simulink model "lab2_pogonya_2018b"  (R2018b)
settings: Solver=FixedStepAuto  StartTime=0.0  StopTime=80  FixedStep=0.05  RelTol=1e-3
settings Model: Creator=User  LastModifiedBy=Танечка
settings DebuggingCC: LibraryContextMissingDiagnostic=none
settings SFSimCC: SimUseLocalCustomCode=off
settings RTWCC: RTWUseLocalCustomCode=off

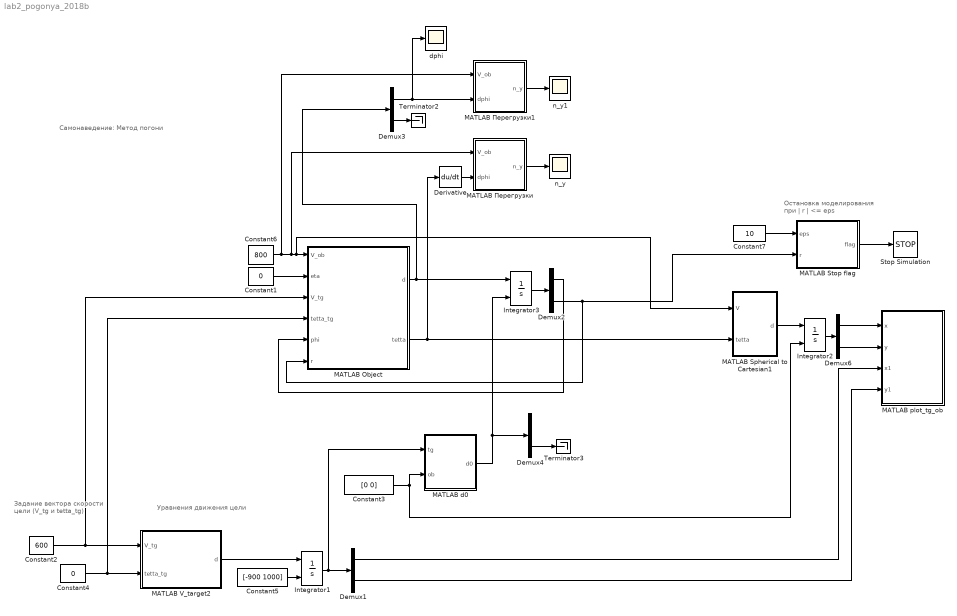
== system lab2_pogonya_2018b ==
  note: Самонаведение: Метод погони
  note: Задание вектора
      | скорости цели
      | (V_tg и tetta_tg)
  note: Остановка моделирования
      | при | r | <= eps
  note: Уравнения
      | движения цели
  Constant1 : Constant  Value=0
  Constant2 : Constant  Value=600
  Constant3 : Constant  Value=[0 0]  VectorParams1D=off
  Constant4 : Constant  Value=0
  Constant5 : Constant  Value=[-900 1000]  VectorParams1D=off
  Constant6 : Constant  Value=800
  Constant7 : Constant  Value=10
  Demux{1..4,6} (5 alike) : Demux  Outputs=2
  Derivative : Derivative
  Integrator1 : Integrator  InitialConditionSource=external
  Integrator2 : Integrator  InitialConditionSource=external
  Integrator3 : Integrator  InitialConditionSource=external
  MATLAB Object : MATLAB Function  TreatAsAtomicUnit=on
  MATLAB Spherical to Cartesian1 : MATLAB Function  TreatAsAtomicUnit=on
  MATLAB Stop flag : MATLAB Function  TreatAsAtomicUnit=on
  MATLAB V_target2 : MATLAB Function  TreatAsAtomicUnit=on
  MATLAB d0 : MATLAB Function  TreatAsAtomicUnit=on
  MATLAB plot_tg_ob : MATLAB Function  TreatAsAtomicUnit=on
  MATLAB Перегрузки : MATLAB Function  TreatAsAtomicUnit=on
  MATLAB Перегрузки1 : MATLAB Function  TreatAsAtomicUnit=on
  Stop Simulation : Stop
  Terminator2 : Terminator
  Terminator3 : Terminator
  dphi : Scope
  n_y : Scope
  n_y1 : Scope
  wires:
  Constant7/1 -> MATLAB Stop flag/1(eps)
  Constant6/1 -> MATLAB Перегрузки1/1(V_ob), MATLAB Spherical to Cartesian1/1(V), MATLAB Object/1(V_ob), MATLAB Перегрузки/1(V_ob)
  MATLAB Object/1(d) -> Integrator3/1, Demux3/1
  MATLAB Stop flag/1(flag) -> Stop Simulation/1
  Integrator3/1 -> Demux2/1
  Demux2/2 -> MATLAB Object/6(r), MATLAB Stop flag/2(r)
  Constant1/1 -> MATLAB Object/2(eta)
  MATLAB Object/2(tetta) -> MATLAB Spherical to Cartesian1/2(tetta), Derivative/1
  Derivative/1 -> MATLAB Перегрузки/2(dphi)
  Constant4/1 -> MATLAB Object/4(tetta_tg), MATLAB V_target2/2(tetta_tg)
  Constant2/1 -> MATLAB Object/3(V_tg), MATLAB V_target2/1(V_tg)
  Constant5/1 -> Integrator1/2
  Integrator1/1 -> Demux1/1, MATLAB d0/1(tg)
  MATLAB V_target2/1(d) -> Integrator1/1
  Demux1/1 -> MATLAB plot_tg_ob/3(x1)
  Demux1/2 -> MATLAB plot_tg_ob/4(y1)
  MATLAB d0/1(d0) -> Integrator3/2, Demux4/1
  Demux2/1 -> MATLAB Object/5(phi)
  Demux3/1 -> MATLAB Перегрузки1/2(dphi), dphi/1
  MATLAB Перегрузки/1(n_y) -> n_y/1
  MATLAB Перегрузки1/1(n_y) -> n_y1/1
  Demux6/1 -> MATLAB plot_tg_ob/1(x)
  Demux6/2 -> MATLAB plot_tg_ob/2(y)
  Constant3/1 -> Integrator2/2, MATLAB d0/2(ob)
  MATLAB Spherical to Cartesian1/1(d) -> Integrator2/1
  Integrator2/1 -> Demux6/1
  Demux3/2 -> Terminator2/1
  Demux4/2 -> Terminator3/1

== matlab function lab2_pogonya_2018b/MATLAB V_target2 ==
  data: V_tg input; tetta_tg input; d output
function d   = func(V_tg, tetta_tg)

dx = V_tg*cos(tetta_tg); 
dy = V_tg*sin(tetta_tg);

d = [dx; dy];

end

== matlab function lab2_pogonya_2018b/MATLAB Перегрузки1 ==
  data: V_ob input; dphi input; n_y output
function n_y  = func( V_ob, dphi)

g = 9.81;

n_y = V_ob*dphi/g;


end

== matlab function lab2_pogonya_2018b/MATLAB d0 ==
  data: tg input; ob input; d0 output
function   d0 = diff( tg, ob)

 x = tg(1) - ob(1);
 y = tg(2) - ob(2);

 phi_0 = atan(y/x); 
 r_0   = sqrt(x^2 + y^2);
   
 d0 = [phi_0; r_0];

end

== matlab function lab2_pogonya_2018b/MATLAB Spherical to Cartesian1 ==
  data: V input; tetta input; d output
function d = func(V, tetta)

% Из сферической системе координат в декартову

    dx = V*cos(tetta);
    dy = V*sin(tetta);             

    d = [dx, dy];

end

== matlab function lab2_pogonya_2018b/MATLAB Перегрузки ==
  data: V_ob input; dphi input; n_y output
function n_y  = func( V_ob, dphi)

g = 9.81;

n_y = V_ob*dphi/g;


end

== matlab function lab2_pogonya_2018b/MATLAB Object ==
  data: d output; V_ob input; eta input; V_tg input; tetta_tg input; phi input; r input; tetta output
function [d, tetta] = Object(V_ob, eta, V_tg, tetta_tg, phi, r)
    tetta = phi - eta;

    dr    =  -V_ob*cos(phi - tetta) + V_tg*cos(phi - tetta_tg);
    dphi  = V_ob*sin(phi - tetta)/r - V_tg*sin(phi - tetta_tg)/r;
%     dphi = phi;

    d = [dphi; dr];
end

== matlab function lab2_pogonya_2018b/MATLAB plot_tg_ob ==
  data: x input; y input; x1 input; y1 input
function plot2d(x,y, x1, y1)

figure(3);
plot(x,y,'ob');
hold on;
plot(x1,y1,'or');
hold on;

xlabel('X');
ylabel('Y');


grid on;
grid minor;
axis('equal');
end

== matlab function lab2_pogonya_2018b/MATLAB Stop flag ==
  data: eps input; r input; flag output
function flag  = Stop_flag(eps, r)

flag = 0;

if abs(r) < eps
          flag = 1;          
end
     
end
